simulink model "GFLIB_VectorLimit_BAM_F32"  (Simulink 8.3)
settings: Solver=ode45  StartTime=0.0  StopTime=10.0  RelTol=1e-3
undefined symbols (not defined in the file): f32Limit
settings Model: Creator=B17364  LastModifiedBy=B17364
settings OptimizationCC: ExpressionDepthLimit=2147483647
settings DebuggingCC: FcnCallInpInsideContextMsg=UseLocalSettings  StrictBusMsg=Warning

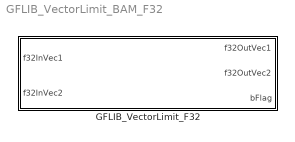
== system GFLIB_VectorLimit_BAM_F32 ==
  GFLIB_VectorLimit_F32 : Subsystem  mask(GFLIB_VectorLimit){f32Limit=f32Limit}
      mask help: Bit accurate model of the GFLIB_VectorLimit function.
      mask init:
      | pos = get_param(gcb, 'Position');width = pos(3) - pos(1); height = pos(4) - pos(2);tX=width/2;tY=height*0.9;
      mask Display: color('black');port_label('input',1,'f32InVec1');port_label('input',2,'f32InVec2');port_label('output',1,'f32OutVec1');port_label('output',2,'f32OutVec2');port_label('output',3,'bFlag');color('black');disp('GFLIB_VectorLimit_F32');color('blue');text(tX,tY, 'BAM', 'horizontalAlignment', 'center');

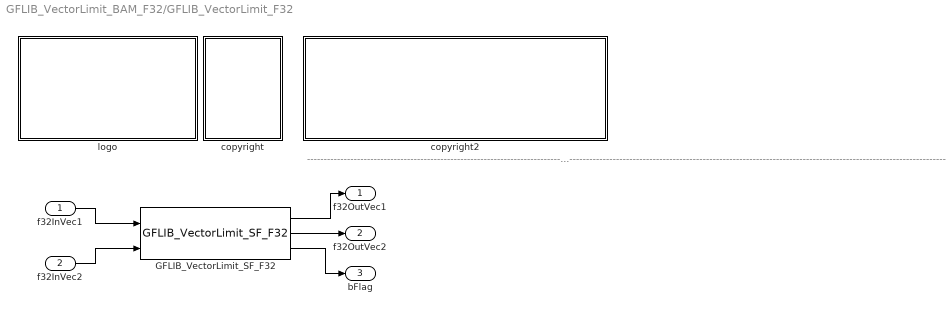
== system GFLIB_VectorLimit_BAM_F32/GFLIB_VectorLimit_F32 ==
  note: ---------------------------------------------------------------------------------------------------------------------------------------------------------------------------------------------------
  f32InVec1 : Inport
  f32InVec2 : Inport  Port=2
  GFLIB_VectorLimit_SF_F32 : S-Function  FunctionName=GFLIB_VectorLimit_SF_F32  Parameters=f32Limit  EnableBusSupport=off
  copyright : Subsystem
      mask Display:
      | text(10,90,'FILE:');text(10,75,'DESRIPTION:')
      | text(10,60,'COPYRIGHT:')
      | text(10,45,'VERSION:')
      | text(10,30,'DATE:')
      | text(10,15,'AUTHOR:')
  copyright2 : Subsystem
      mask Display:
      | text(10,90,'GFLIB_VectorLimit_BAM_F32.mdl');text(10,75,'Vector limit function');text(10,60,'Freescale')
      | text(10,45,'0.1');text(10,30,'15-Sep-2011');text(10,15,'');
  logo : Subsystem
      mask Display: image(imread('logo.jpg'))
  f32OutVec1 : Outport
  f32OutVec2 : Outport  Port=2
  bFlag : Outport  Port=3
  wires:
  f32InVec1/1 -> GFLIB_VectorLimit_SF_F32/1
  GFLIB_VectorLimit_SF_F32/1 -> f32OutVec1/1
  f32InVec2/1 -> GFLIB_VectorLimit_SF_F32/2
  GFLIB_VectorLimit_SF_F32/2 -> f32OutVec2/1
  GFLIB_VectorLimit_SF_F32/3 -> bFlag/1

== system GFLIB_VectorLimit_BAM_F32/GFLIB_VectorLimit_F32/copyright ==

== system GFLIB_VectorLimit_BAM_F32/GFLIB_VectorLimit_F32/copyright2 ==

== system GFLIB_VectorLimit_BAM_F32/GFLIB_VectorLimit_F32/logo ==
